simulink library "bcm"  (R2021b)
settings: Solver=VariableStepAuto  StartTime=0.0  StopTime=10.0  RelTol=1e-3
undefined symbols (not defined in the file): ENUM_ANTITHEFT_ALARM, ENUM_ANTITHEFT_ARM, ENUM_ANTITHEFT_DISARM, ENUM_ANTITHEFT_WAIT, ENUM_GEARPOSNTOCAN_P, ENUM_PDKEYRAWLULOCK_INUNLOCK, ENUM_PDKEYRAWPS_INPS, ENUM_POWERSTA_ON, ENUM_POWERSTA_READY, ENUM_POWERSTA_STANDBY, ENUM_PWRSTASW_ON, ENUM_PWRSTASW_READY, ENUM_SYSMODE_DEVELOPING, ENUM_SYSMODE_PRODUCT, ENUM_VEHICLETYPE_D21, ENUM_VEHICLETYPE_D31F25, ENUM_VEHICLETYPE_D31HAWD, ENUM_VEHICLETYPE_D31HRWD, ENUM_VEHICLETYPE_D31L24, FALSE, KBCM_ACCSwcPrsTmr_s, KBCM_ALMBrightnessDark_enum, KBCM_AmbBlue_enum, KBCM_AmbBreathT_ms, KBCM_AmbGreen_enum, KBCM_AmbMidPple_enum, KBCM_AmbRed_enum, KBCM_AmbTempCtrlEN_flg, KBCM_AmbTempT_s, KBCM_AmbWelModeENWait_s, KBCM_Antitheft_enum_ovrdflg, KBCM_Antitheft_enum_ovrdval, KBCM_APMDoorCtrlSta_flg_ovrdflg, KBCM_APMDoorCtrlSta_flg_ovrdval, KBCM_CmdKeepT_s, KBCM_CSWLightRstDebT_s, KBCM_CSWTurnLPRstT_s, KBCM_CycleTimeSet_s, KBCM_DelayTSW_flg, KBCM_DiagDRLOFF_flg, KBCM_DiagFLTC_mA, KBCM_DiagFMHT_s, KBCM_DiagFRTC_mA, KBCM_DiagRLTC_mA, KBCM_DiagRRTC_mA, KBCM_DrAPMRetryTimes_cnt, KBCM_DrOpenWdwOT_s, KBCM_DrOpenWdwReady_s, KBCM_DutyCycleSet_cnt, KBCM_DutyOverride_flg, KBCM_DutyOverride_val, KBCM_ESSOffT_ms, KBCM_ESSOnT_ms, KBCM_FDCDKCReDetectT_K, KBCM_FDCDKCUSSFilterT_K, KBCM_HandleLampKeepT_s, KBCM_IVIRstHoldT_ms, KBCM_IVIRstTriggerT_ms, KBCM_ONDelayT_ms, KBCM_RAPSAbnFlashOFFT_ms ... (+51)
libraries: simulink x402, $bdroot x10, hcu_lib x2
(part 14 of 14)

== stateflow chart bcm/BCM/BCM/PTG/Chart ==
  state Alarm
    en:
    VBCM_SPTGDet_flg=1;
  state NoDetected
    en:
    VBCM_SPTGDet_flg=0;
    VBCM_APSOpenPTG_flg=0;
  state WaitForDKC
  state DoorOpen
    en:
    VBCM_SPTGDet_flg=0;
    VBCM_APSOpenPTG_flg=1;
  state WaitforLeave
    en:
    VBCM_APSOpenPTG_flg=0;
    VBCM_SPTGDet_flg=0;
    state OutRange
    state InRange
    (default) -> InRange
    InRange -> OutRange : [(PASDRMR>=100 || PASDRML>=100) && (!TailgateSW)]
    OutRange -> InRange [order 1] : [(PASDRMR<100 && PASDRML<100) || TailgateSW]
  (junction 109) -> NoDetected [order 1] : [KBCM_DelayTSW_flg==0]{VBCM_u8DetectWaitT_s=0;}
  Alarm -> (junction 109) [order 1] : [hasChangedTo(KeyDetectedOut,0)....
      | &&....
      | KBCM_SPTGLeave_flg==1]
  (junction 109) -> (junction 70) [order 2]
  (junction 70) -> NoDetected : {VBCM_u8DetectWaitT_s=KBCM_SPTGDetectWaitT_s;}
  (junction 128) -> Alarm
  WaitForDKC -> (junction 128) [order 1] : [PDKeyAreaPTG==1]
  NoDetected -> NoDetected [order 2] : [VBCM_u8DetectWaitT_s>0]{VBCM_u8DetectWaitT_s=VBCM_u8DetectWaitT_s-1;}
  Alarm -> WaitforLeave [order 2] : [ShiftGearPosn!=0||....
      | VehSpeed>0||....
      | PwrSta==5||....
      | TailgateSW!=0||....
      | IVI_PTG_USSta_SW!=0||....
      | PDKeyAreaPTG!=1]
  Alarm -> WaitforLeave [order 3] : [DKCKeyPress]
  Alarm -> DoorOpen [order 4] : [after(KBCM_SPTGDetectT_sec*100,tick)]
  NoDetected -> WaitForDKC [order 1] : [hasChangedTo(KeyDetected,1)&&VBCM_u8DetectWaitT_s==0....
      | &&....
      | (ShiftGearPosn==0&&....
      | VehSpeed<=0&&....
      | PwrSta!=5&&....
      | TailgateSW==0&&....
      | IVI_PTG_USSta_SW==0)]
  DoorOpen -> WaitforLeave : [after(40,tick)]
  (default) -> WaitforLeave
  (junction 136) -> NoDetected [order 1] : [KBCM_DelayTSW_flg==0]{VBCM_u8DetectWaitT_s=0;}
  WaitForDKC -> (junction 136) [order 2] : [hasChangedTo(KeyDetectedOut,0)....
      | &&....
      | KBCM_SPTGLeave_flg==1]
  (junction 136) -> (junction 138) [order 2]
  WaitForDKC -> WaitforLeave [order 3] : [after(KBCM_SPTGWaitDKC_sec*100,tick)]
  (junction 138) -> NoDetected : {VBCM_u8DetectWaitT_s=100;}
  OutRange -> NoDetected [order 2] : after(KBCM_ReDetectT_K,tick)
  data: KBCM_DelayTSW_flg input; KeyDetected input; PASDRMR input; PASDRML input; PDKeyAreaPTG input; PwrSta input; KeyDetectedOut input; TailgateSW input; VehSpeed input; DKCKeyPress input; ShiftGearPosn input; IVI_PTG_USSta_SW input; VBCM_APSOpenPTG_flg output; VBCM_SPTGDet_flg output; VBCM_u8DetectWaitT_s local uint8 =0; KBCM_ReDetectT_K input =1; KBCM_SPTGDetectT_sec input; KBCM_SPTGLeave_flg input; KBCM_SPTGWaitDKC_sec input; KBCM_SPTGDetectWaitT_s input

== stateflow chart bcm/BCM/BCM/APM_Door/DoorAPM/window ==
  state Normal
    state DoorClose
      state NoResponse
      state PwrOpenReq
        en:CtrlCmd = 126;
      state WinClose
        en:CtrlCmd = 0;
        ex:CtrlCmd = 127;
      state StandBy
      (default) -> (junction 123)
      (junction 123) -> (junction 124) [order 1] : [ Val_Wdw_Opened > 8....
          | ||....
          | Val_Wdw_Opened <= 0 ]
      (junction 123) -> (junction 58) [order 2]
      (junction 124) -> Normal.DoorClose.NoResponse
      (junction 58) -> (junction 56) [order 1] : [!CANMsgValidGWZoneDR1....
          | ||....
          | !CANMsgValidGWZoneFR1]
      (junction 56) -> Normal.DoorClose.NoResponse [order 2]
      (junction 58) -> WinClose [order 2]
      (junction 56) -> Normal.DoorClose.PwrOpenReq [order 1] : [DrAPMRetryCnt<KBCM_DrAPMRetryTimes_cnt]
      (junction 130) -> Normal.DoorClose.NoResponse
      Normal.DoorClose.PwrOpenReq -> WinClose [order 1] : [CANMsgValidGWZoneDR1....
          | &&....
          | CANMsgValidGWZoneFR1]
      WinClose -> Normal.DoorClose.StandBy : [Val_Wdw_Opened <= 0 || ...
          | after(DrOpenWdwOT_K,tick)]
      Normal.DoorClose.PwrOpenReq -> (junction 99) [order 2]
      (junction 99) -> Normal.DoorClose.StandBy : [after(WaitAPMPwr_K,tick)]
          | {CtrlCmd=127;
          | DrAPMRetryCnt=DrAPMRetryCnt+1;}
      Normal.DoorClose.StandBy -> (junction 130) [order 1] : [hasChanged(Val_Wdw_Opened)]
    state DoorOpen
      state NoResponse
      state WinOpen
        en:CtrlCmd = 6;
        ex:CtrlCmd = 127;
      state PwrOpenReq
        en:CtrlCmd = 126;
      state StandBy
      (default) -> (junction 48)
      (junction 48) -> (junction 120) [order 1]
      (junction 48) -> (junction 51) [order 2] : [!CANMsgValidGWZoneDR1....
          | ||....
          | !CANMsgValidGWZoneFR1]
      (junction 51) -> Normal.DoorOpen.NoResponse [order 2]
      (junction 120) -> Normal.DoorOpen.StandBy : [ Val_Wdw_Opened > 0 ]
      (junction 48) -> WinOpen [order 3]
      (junction 51) -> Normal.DoorOpen.PwrOpenReq [order 1] : [DrAPMRetryCnt<KBCM_DrAPMRetryTimes_cnt]
      Normal.DoorOpen.PwrOpenReq -> WinOpen [order 1] : [CANMsgValidGWZoneDR1....
          | &&....
          | CANMsgValidGWZoneFR1]
      Normal.DoorOpen.PwrOpenReq -> (junction 102) [order 2]
      WinOpen -> Normal.DoorOpen.StandBy : [Val_Wdw_Opened >= 6 || ...
          | after(DrOpenWdwOT_K,tick)]
      (junction 102) -> Normal.DoorOpen.StandBy : [after(WaitAPMPwr_K,tick)]
          | {CtrlCmd=127;
          | DrAPMRetryCnt=DrAPMRetryCnt+1;}
    state Reverse
    (default) -> DoorClose
    (junction 8) -> DoorClose [order 1] : [!DoorSW]
    (junction 8) -> DoorOpen [order 2]
    Reverse -> (junction 8) : [CtrlCmd_Ready]
    (junction 21) -> Reverse [order 2]
    DoorClose -> (junction 21) : [DoorSW]
        | {DrAPMRetryCnt=0;}
    (junction 21) -> DoorOpen [order 1] : [CtrlCmd_Ready]
    (junction 29) -> (junction 21) [order 2]
    (junction 29) -> DoorClose [order 1] : [CtrlCmd_Ready]
    DoorOpen -> (junction 29) : [!DoorSW]
        | {DrAPMRetryCnt=0;}
    (junction 94) -> (junction 29)
    Normal.DoorClose.StandBy -> (junction 94) [order 2] : [ Val_Wdw_Opened <= 8 && Val_Wdw_Opened > 0 ]
    Normal.DoorOpen.StandBy -> (junction 94) [order 2] : [ Val_Wdw_Opened <= 0 ]
  state ManualOpen
    en:
    CtrlCmd = 127;
  state IVICmdSend
    en:
    CtrlCmd = ControlCommand_Buf;
  state CommandRst
    en:
    CtrlCmd=127;
  (default) -> ManualOpen
  ManualOpen -> (junction 65) [order 2]
  Normal -> (junction 65) [order 1]
  (junction 65) -> (junction 66) : [hasChangedFrom(ControlCommand, 127)]
      | {ControlCommand_Buf = ControlCommand;}
  (junction 66) -> (junction 79) [order 2]
  (junction 79) -> IVICmdSend
  (junction 66) -> CommandRst [order 1] : [!CtrlCmd_Ready]
  CommandRst -> IVICmdSend : [CtrlCmd_Ready]
  IVICmdSend -> ManualOpen : [after(12,tick)]
  Normal -> ManualOpen [order 2] : [!APMDoorControlSta]
  ManualOpen -> Normal.DoorClose.StandBy [order 1] : [APMDoorControlSta]
      | {DrAPMRetryCnt=0;}
  Normal.DoorOpen.StandBy -> ManualOpen [order 1] : [( hasChanged(Val_Wdw_Opened) && ( Val_Wdw_Opened>=8 ) ) && after(KBCM_WdwManualDetT_K,tick)]
  data: DoorSW input boolean; Val_Wdw_Opened input uint8; WaitAPMPwr_K input uint8; APMDoorControlSta input; CtrlCmd_Ready input; ControlCommand input; DrOpenWdwOT_K input uint8; CtrlCmd output uint8; ControlCommand_Buf local uint8; KBCM_WdwManualDetT_K input; CANMsgValidGWZoneDR1 input boolean; CANMsgValidGWZoneFR1 input boolean; KBCM_DrAPMRetryTimes_cnt input; DrAPMRetryCnt local uint8 =0

== stateflow chart bcm/BCM/BCM/Personal_Setting/ACC/Chart ==
  state ACC_Disable
    en:
    VBCM_LRightStaCmd_flg = VINP_SWC2LRightSta_flg;
    VBCM_LLeftStaCmd_flg = VINP_SWC2LLeftSta_flg;
    VBCM_ACCSetUpCnt_cnt = 0;
    VBCM_ACCSetDnCnt_cnt = 0;
    du:
    VBCM_LRightStaCmd_flg = VINP_SWC2LRightSta_flg;
    VBCM_LLeftStaCmd_flg = VINP_SWC2LLeftSta_flg;
  state ACC_Sync
    en:
    VBCM_LRightStaCmd_flg = 0;
    VBCM_LLeftStaCmd_flg = 0;
  state UP_Press
    en:
    VBCM_LRightStaCmd_flg = 1;
    VBCM_LLeftStaCmd_flg = 0;
  state DN_Press
    en:
    en:
    VBCM_LRightStaCmd_flg = 0;
    VBCM_LLeftStaCmd_flg = 1;
  state ACC_Enable
    en:
    VBCM_LRightStaCmd_flg = 0;
    VBCM_LLeftStaCmd_flg = 0;
    du:
    VBCM_LRightStaCmd_flg = 0;
    VBCM_LLeftStaCmd_flg = 0;
  (default) -> ACC_Disable
  ACC_Sync -> ACC_Disable [order 1] : [!VBCM_ACCChangeEnable_flg]
  ACC_Sync -> UP_Press [order 2] : [after(KBCM_ACCSwcPrsTmr_s,tick)....
      | &&....
      | VBCM_ACCSetUpCnt_cnt > 0]
      | {VBCM_ACCSetUpCnt_cnt = VBCM_ACCSetUpCnt_cnt -1;}
  UP_Press -> ACC_Sync : [after(KBCM_ACCSwcPrsTmr_s,tick)]
  DN_Press -> ACC_Sync : [after(KBCM_ACCSwcPrsTmr_s,tick)]
  ACC_Sync -> DN_Press [order 3] : [after(KBCM_ACCSwcPrsTmr_s,tick)&&....
      | VBCM_ACCSetDnCnt_cnt > 0]
      | {VBCM_ACCSetDnCnt_cnt = VBCM_ACCSetDnCnt_cnt -1;}
  ACC_Sync -> ACC_Enable [order 4] : [VBCM_ACCSetUpCnt_cnt == 0....
      | &&....
      | VBCM_ACCSetDnCnt_cnt == 0....
      | &&....
      | after(KBCM_WaitACCChange_s,tick)]
  ACC_Enable -> ACC_Sync [order 2] : [VINP_TimeGapLevel_enum <= 4 && VINP_TimeGapLevel_enum > VBCM_TimeGapLevelSta_enum]
      | {VBCM_ACCSetUpCnt_cnt = 0;
      |  VBCM_ACCSetDnCnt_cnt = VINP_TimeGapLevel_enum - VBCM_TimeGapLevelSta_enum;}
  ACC_Enable -> ACC_Sync [order 3] : [VINP_TimeGapLevel_enum <= 4 && VINP_TimeGapLevel_enum < VBCM_TimeGapLevelSta_enum]
      | {VBCM_ACCSetUpCnt_cnt = VBCM_TimeGapLevelSta_enum - VINP_TimeGapLevel_enum;....
      |  VBCM_ACCSetDnCnt_cnt = 0;}
  ACC_Disable -> ACC_Enable : [VBCM_ACCChangeEnable_flg]
  ACC_Enable -> ACC_Disable [order 1] : [!VBCM_ACCChangeEnable_flg]
  data: VBCM_ACCChangeEnable_flg input; VBCM_LRightStaCmd_flg output boolean; VBCM_LLeftStaCmd_flg output boolean; VINP_TimeGapLevel_enum input; VBCM_TimeGapLevelSta_enum input; VINP_SWC2LRightSta_flg input; VINP_SWC2LLeftSta_flg input; VBCM_ACCSetDnCnt_cnt local uint8; VBCM_ACCSetUpCnt_cnt local uint8; KBCM_ACCSwcPrsTmr_s input; KBCM_WaitACCChange_s input

== stateflow chart bcm/BCM/BCM/CSW/Chart ==
  state OFF
    en:CSW2TSw=0;
  state LeftControl
    en:CSW2TSw=1;
    state LightLeft
      state Debounce
      state Hold
      state StandBy
      (default) -> LeftControl.LightLeft.StandBy
      LeftControl.LightLeft.StandBy -> LeftControl.LightLeft.Debounce [order 1] : [hasChanged(VINP_CSW2TurnSwSta_enum) &&....
          | VINP_CSW2TurnSwSta_enum == 3]
      LeftControl.LightLeft.StandBy -> LeftControl.LightLeft.Hold [order 2] : [after(tset,tick) ||....
          | hasChanged(VINP_CSW2TurnSwSta_enum) &&....
          | VINP_CSW2TurnSwSta_enum == 1]
    state Left
      state Debounce
      state StandBy
      (default) -> LeftControl.Left.StandBy
      LeftControl.Left.StandBy -> LeftControl.Left.Debounce [order 1] : [hasChanged(VINP_CSW2TurnSwSta_enum) &&....
          | VINP_CSW2TurnSwSta_enum == 3]
      LeftControl.Left.StandBy -> (junction 119) [order 2] : [hasChanged(VINP_CSW2TurnSwSta_enum) &&....
          | VINP_CSW2TurnSwSta_enum == 1]
    (default) -> LightLeft
    (junction 119) -> LeftControl.LightLeft.Hold
    LightLeft -> Left : [VINP_CSW2TurnSwSta_enum == 2]
  state RESET
    en:CSW2TSw = 0;
  state RightControl
    en:CSW2TSw=2;
    state Right
      state Debounce
      state StandBy
      (default) -> RightControl.Right.StandBy
      RightControl.Right.StandBy -> RightControl.Right.Debounce [order 1] : [hasChanged(VINP_CSW2TurnSwSta_enum) &&....
          | VINP_CSW2TurnSwSta_enum == 1]
      RightControl.Right.StandBy -> (junction 153) [order 2] : [hasChanged(VINP_CSW2TurnSwSta_enum) &&....
          | VINP_CSW2TurnSwSta_enum == 3]
    state LightRight
      state Hold
      state Debounce
      state StandBy
      (default) -> RightControl.LightRight.StandBy
      RightControl.LightRight.StandBy -> RightControl.LightRight.Debounce [order 1] : [hasChanged(VINP_CSW2TurnSwSta_enum) &&....
          | VINP_CSW2TurnSwSta_enum == 1]
      RightControl.LightRight.StandBy -> RightControl.LightRight.Hold [order 2] : [after(tset,tick) ||....
          | hasChanged(VINP_CSW2TurnSwSta_enum) &&....
          | VINP_CSW2TurnSwSta_enum == 3]
    (junction 153) -> RightControl.LightRight.Hold
    LightRight -> Right : [VINP_CSW2TurnSwSta_enum == 4 ]
    (default) -> LightRight
  (default) -> OFF
  LeftControl.LightLeft.Debounce -> OFF [order 1] : [VINP_CSW2TurnSwSta_enum != 3 && VINP_CSW2TurnSwSta_enum != 4]
  OFF -> (junction 110) [order 1] : [VINP_CSW2TurnSwSta_enum == 1]
  (junction 110) -> LeftControl [order 1] : [hasChanged(VINP_CSW2TurnSwSta_enum)]
  (junction 110) -> (junction 113) [order 2]
  (junction 113) -> LeftControl.LightLeft.Hold
  LeftControl.LightLeft.Debounce -> RESET [order 2] : [after(KBCM_CSWLightRstDebT_s,tick)]
  LeftControl.LightLeft.Hold -> OFF : [VINP_CSW2TurnSwSta_enum != 1]
  OFF -> Left [order 2] : [VINP_CSW2TurnSwSta_enum == 2]
  Left -> OFF : [LeftRelflg && VINP_CSW2TurnSwSta_enum != 1 && VINP_CSW2TurnSwSta_enum != 2]
  LeftControl.Left.Debounce -> OFF [order 1] : [VINP_CSW2TurnSwSta_enum != 3 && VINP_CSW2TurnSwSta_enum != 4]
  LeftControl.Left.Debounce -> RESET [order 2] : [after(KBCM_CSWLightRstDebT_s,tick)]
  RightControl -> LeftControl : [VINP_CSW2TurnSwSta_enum == 2]
  LeftControl -> RightControl : [VINP_CSW2TurnSwSta_enum == 4]
  RESET -> OFF : [ (VINP_CSW2TurnSwSta_enum != 1 && VINP_CSW2TurnSwSta_enum != 3) || after(KBCM_CSWTurnLPRstT_s,tick)]
  RightControl.Right.Debounce -> RESET [order 1] : [after(KBCM_CSWLightRstDebT_s,tick)]
  RightControl.LightRight.Debounce -> RESET [order 1] : [after(KBCM_CSWLightRstDebT_s,tick)]
  RightControl.Right.Debounce -> OFF [order 2] : [VINP_CSW2TurnSwSta_enum != 1 && VINP_CSW2TurnSwSta_enum != 2]
  OFF -> Right [order 4] : [ VINP_CSW2TurnSwSta_enum == 4 ]
  Right -> OFF : [ RightRelflg && VINP_CSW2TurnSwSta_enum != 3 && VINP_CSW2TurnSwSta_enum != 4 ]
  OFF -> (junction 183) [order 3] : [VINP_CSW2TurnSwSta_enum == 3]
  (junction 183) -> RightControl [order 1] : [hasChanged(VINP_CSW2TurnSwSta_enum)]
  (junction 183) -> (junction 179) [order 2]
  (junction 179) -> RightControl.LightRight.Hold
  RightControl.LightRight.Hold -> OFF : [ VINP_CSW2TurnSwSta_enum != 3 ]
  RightControl.LightRight.Debounce -> OFF [order 2] : [ VINP_CSW2TurnSwSta_enum != 1 && VINP_CSW2TurnSwSta_enum != 2 ]
  data: VINP_CSW2TurnSwSta_enum input uint8; LeftRelflg input boolean; RightRelflg input boolean; CSW2TSw output uint8; tset input uint16; KBCM_CSWLightRstDebT_s input; KBCM_CSWTurnLPRstT_s input

== stateflow chart bcm/BCM/BCM/FlasherSignal/flasher1/Chart ==
  state init
    en:
    time_cnt = ZERO_INT;
    ON_flg = FALSE;
    OFF_flg = FALSE;
    out = FALSE;
    CycleCnt_cnt = ZERO_INT;
  state OFF
    en:
    out = FALSE;
    time_cnt = ZERO_INT;
    OFF -> (junction 38) [order 1]
    (junction 38) -> OFF : {time_cnt = time_cnt + ONE_INT;}
  state ON
    en:
    out = TRUE;
    time_cnt = ZERO_INT;
    du:
    time_cnt = time_cnt +ONE_INT;
  state WAIT
    en:
    out = FALSE;
    time_cnt = ZERO_INT;
    du:
    time_cnt = time_cnt + ONE_INT;
  (default) -> init
  (junction 73) -> (junction 74)
  (junction 74) -> init
  (junction 70) -> init
  (junction 75) -> (junction 73)
  OFF -> (junction 74) [order 1] : [~Trig_flg]
  ON -> (junction 70) [order 1] : [~Trig_flg]
  init -> (junction 57) : [Trig_flg]
  (junction 57) -> ON : {ON_flg = TRUE;}
  OFF -> (junction 46) [order 3] : [time_cnt > OFF_cnt]
  (junction 46) -> (junction 47) : {time_cnt = ZERO_INT; ON_flg = TRUE; OFF_flg = FALSE; CycleCnt_cnt = CycleCnt_cnt +ONE_INT;}
  (junction 47) -> ON : [ON_flg]
  ON -> (junction 44) [order 2] : [time_cnt > ON_cnt]
  (junction 44) -> (junction 42) : {time_cnt = ZERO_INT; ON_flg = FALSE; OFF_flg = TRUE;}
  (junction 42) -> OFF : [OFF_flg]
  OFF -> (junction 66) [order 2] : [time_cnt > OFF_cnt && CycleCnt_cnt >= Cycle_cnt]
  (junction 66) -> WAIT : {time_cnt = ZERO_INT;}
  (junction 62) -> ON : {time_cnt = ZERO_INT; ON_flg = TRUE; OFF_flg = FALSE; CycleCnt_cnt = ZERO_INT;}
  WAIT -> (junction 62) [order 2] : [time_cnt >= WAIT_cnt]
  WAIT -> (junction 75) [order 1] : [~Trig_flg]
  data: ON_cnt input; OFF_cnt input; WAIT_cnt input; Cycle_cnt input; out output boolean; time_cnt local uint8; OFF_flg local boolean; ON_flg local boolean; CycleCnt_cnt local uint8; Trig_flg input; FALSE parameter; TRUE parameter; ONE_INT parameter; ZERO_INT parameter

== stateflow chart bcm/BCM/BCM/FlasherSignal/flasher/Chart ==
  state init
    en:
    time_cnt = ZERO_INT;
    ON_flg = FALSE;
    OFF_flg = FALSE;
    out = FALSE;
    CycleCnt_cnt = ZERO_INT;
  state OFF
    en:
    out = FALSE;
    time_cnt = ZERO_INT;
    OFF -> (junction 38) [order 1]
    (junction 38) -> OFF : {time_cnt = time_cnt + ONE_INT;}
  state ON
    en:
    out = TRUE;
    time_cnt = ZERO_INT;
    du:
    time_cnt = time_cnt +ONE_INT;
  state WAIT
    en:
    out = FALSE;
    time_cnt = ZERO_INT;
    du:
    time_cnt = time_cnt + ONE_INT;
  (default) -> init
  (junction 73) -> (junction 74)
  (junction 74) -> init
  (junction 70) -> init
  (junction 75) -> (junction 73)
  OFF -> (junction 74) [order 1] : [~Trig_flg]
  ON -> (junction 70) [order 1] : [~Trig_flg]
  init -> (junction 57) : [Trig_flg]
  (junction 57) -> ON : {ON_flg = TRUE;}
  OFF -> (junction 46) [order 3] : [time_cnt > OFF_cnt]
  (junction 46) -> (junction 47) : {time_cnt = ZERO_INT; ON_flg = TRUE; OFF_flg = FALSE; CycleCnt_cnt = CycleCnt_cnt +ONE_INT;}
  (junction 47) -> ON : [ON_flg]
  ON -> (junction 44) [order 2] : [time_cnt > ON_cnt]
  (junction 44) -> (junction 42) : {time_cnt = ZERO_INT; ON_flg = FALSE; OFF_flg = TRUE;}
  (junction 42) -> OFF : [OFF_flg]
  OFF -> (junction 66) [order 2] : [time_cnt > OFF_cnt && CycleCnt_cnt >= Cycle_cnt]
  (junction 66) -> WAIT : {time_cnt = ZERO_INT;}
  (junction 62) -> ON : {time_cnt = ZERO_INT; ON_flg = TRUE; OFF_flg = FALSE; CycleCnt_cnt = ZERO_INT;}
  WAIT -> (junction 62) [order 2] : [time_cnt >= WAIT_cnt]
  WAIT -> (junction 75) [order 1] : [~Trig_flg]
  data: ON_cnt input; OFF_cnt input; WAIT_cnt input; Cycle_cnt input; out output boolean; time_cnt local uint8; OFF_flg local boolean; ON_flg local boolean; CycleCnt_cnt local uint8; Trig_flg input; FALSE parameter; TRUE parameter; ONE_INT parameter; ZERO_INT parameter
